simulink model "p560_jacobiano_ciclico_sp"  (R2020b)
settings: Solver=VariableStepAuto  StartTime=0.0  StopTime=50  RelTol=1e-3
values from neighbouring files (symbols this model uses):
  fr = 1    [init.m]
undefined symbols (not defined in the file or in its folder): DiscIntNeverNeededParam, qn
libraries: roblocks x6
settings Model: Creator=Valentina  LastModifiedBy=Valentina

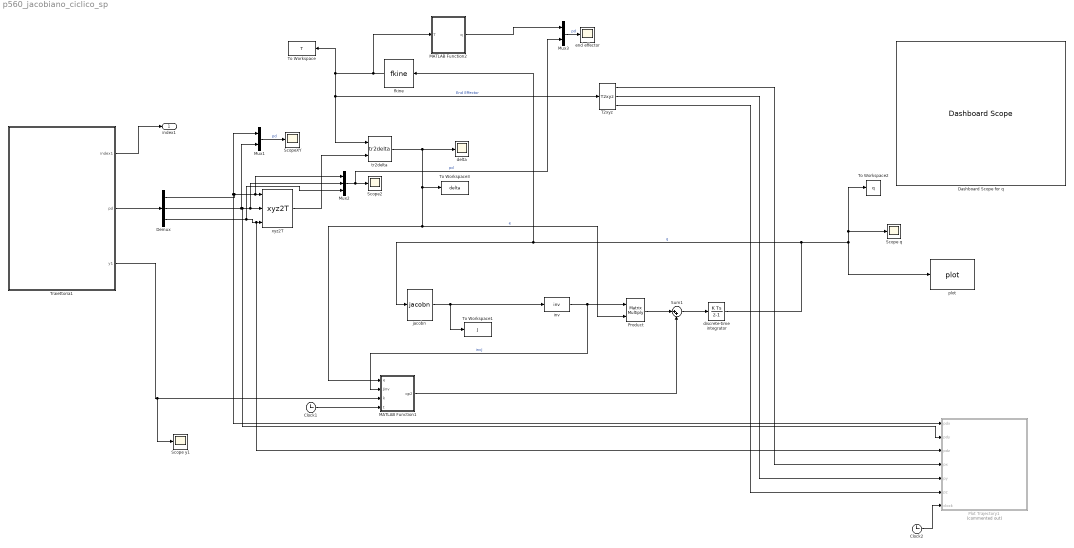
== system p560_jacobiano_ciclico_sp ==
  Clock1 : Clock
  Clock2 : Clock
  Dashboard Scope for q : DashboardScope
  Demux : Demux  Outputs=3
  MATLAB Function1 : MATLAB Function  Priority=6  TreatAsAtomicUnit=on  SystemSampleTime=2*pi/100
  MATLAB Function2 : MATLAB Function  Priority=6  TreatAsAtomicUnit=on
  Mux1 : Mux  Inputs=2
  Mux2 : Mux  Inputs=3
  Mux3 : Mux  Inputs=2
  Plot Trajectory1 : MATLAB Function  Commented=on  TreatAsAtomicUnit=on  SystemSampleTime=0.1
  Product : Product  Multiplication=Matrix(*)  InputSameDT=on  RndMeth=Zero  SaturateOnIntegerOverflow=on  OutDataTypeStr=Inherit: Same as first input
  Scope q : Scope
  Scope y1 : Scope
  Scope2 : Scope
  ScopeXY : Scope
  Sum1 : Sum  Inputs=|++
  T2xyz : roblocks/Toolbox/T2xyz
  To Workspace : ToWorkspace  VariableName=T  SampleTime=-1
  To Workspace1 : ToWorkspace  VariableName=J  SampleTime=-1
  To Workspace2 : ToWorkspace  VariableName=q  SampleTime=-1
  To Workspace3 : ToWorkspace  VariableName=delta  SampleTime=-1
  Traiettoria1 : Subsystem
  delta : Scope
  discrete-time integrator : DiscreteIntegrator  gainval=5  InitialCondition=qn  SampleTime=0.1  ICPrevOutput=DiscIntNeverNeededParam  ICPrevScaledInput=DiscIntNeverNeededParam
  end effector : Scope
  fkine : roblocks/Arm/fkine  robot=p560
  inv : MATLABFcn  MATLABFcn=inv  Output1D=off
  jacobn : roblocks/Arm/jacobn  robot=p560
  plot : roblocks/Arm/plot  robot=p560  fps=5  holdplot=on
  tr2delta : roblocks/Toolbox/tr2delta
  xyz2T : roblocks/Toolbox/xyz2T
  index1 : Outport
  wires:
  T2xyz/3 -> Plot Trajectory1/6(pz)
  Demux/1 -> Mux1/1, Plot Trajectory1/1(pdx), Mux2/1, xyz2T/1
  T2xyz/1 -> Plot Trajectory1/4(px)
  Clock2/1 -> Plot Trajectory1/7(clock)
  fkine/1 -> MATLAB Function2/1(T), To Workspace/1, tr2delta/1, T2xyz/1  "End Effector"
  T2xyz/2 -> Plot Trajectory1/5(py)
  tr2delta/1 -> delta/1, To Workspace3/1, Product/2, MATLAB Function1/1(e)  "e"
  Mux1/1 -> ScopeXY/1  "pd"
  MATLAB Function1/1(qp2) -> Sum1/2
  Demux/2 -> Mux1/2, Plot Trajectory1/2(pdy), Mux2/2, xyz2T/2
  jacobn/1 -> To Workspace1/1, inv/1
  xyz2T/1 -> tr2delta/2
  Sum1/1 -> discrete-time integrator/1
  discrete-time integrator/1 -> fkine/1, jacobn/1, plot/1, Scope q/1, To Workspace2/1  "q"
  Clock1/1 -> MATLAB Function1/4(t)
  inv/1 -> MATLAB Function1/2(Jinv), Product/1  "invJ"
  Product/1 -> Sum1/1
  Demux/3 -> Mux2/3, Plot Trajectory1/3(pdz), xyz2T/3
  Traiettoria1/2(pd) -> Demux/1
  Traiettoria1/1(index1) -> index1/1
  Traiettoria1/3(y1) -> Scope y1/1, MATLAB Function1/3(k)
  Mux2/1 -> Mux3/2, Scope2/1  "pd"
  Mux3/1 -> end effector/1  "pd"
  MATLAB Function2/1(q) -> Mux3/1

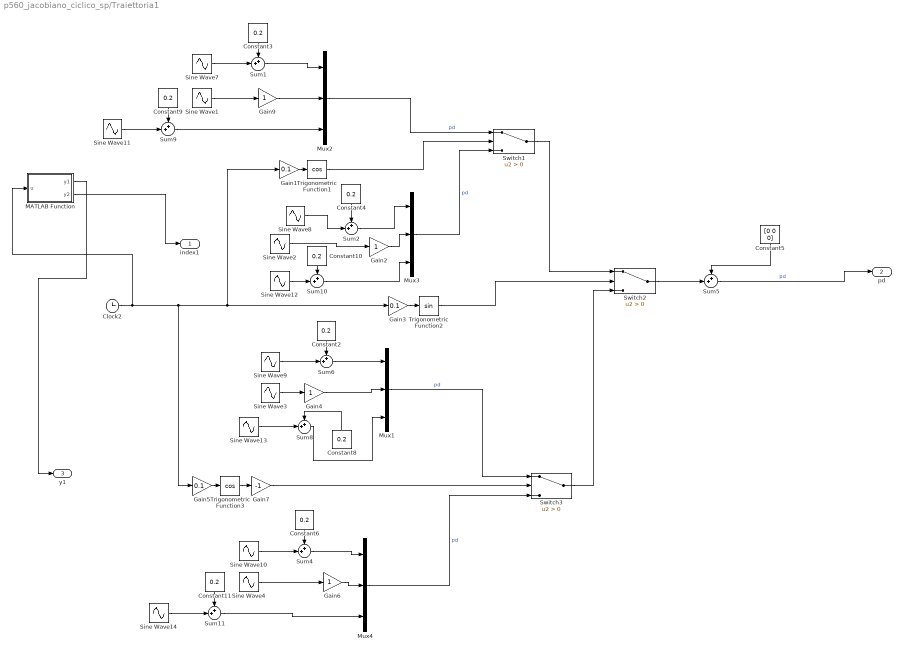
== system p560_jacobiano_ciclico_sp/Traiettoria1 ==
  Clock2 : Clock
  Constant{2..4,6,8..11} (8 alike) : Constant  Value=0.2
  Constant5 : Constant  Value=[0 0 0]
  Gain1 : Gain  Gain=0.1
  Gain{2,4,6,9} (4 alike) : Gain
  Gain3 : Gain  Gain=0.1
  Gain5 : Gain  Gain=0.1
  Gain7 : Gain  Gain=-1
  MATLAB Function : MATLAB Function  TreatAsAtomicUnit=on  SystemSampleTime=2*pi/100
  Mux{1..4} (4 alike) : Mux  Inputs=3
  Sine Wave{1..4} (4 alike) : Sin  Amplitude=0.5  Frequency=fr  Phase=pi/2  SampleTime=0
  Sine Wave{7..10} (4 alike) : Sin  Amplitude=0.5  Frequency=fr  SampleTime=0
  Sine Wave{11..14} (4 alike) : Sin  Amplitude=0.2  Frequency=fr  SampleTime=0
  Sum{1..2,4..6,8..11} (9 alike) : Sum  Inputs=++|
  Switch1 : Switch  Criteria=u2 > Threshold
  Switch2 : Switch  Criteria=u2 > Threshold
  Switch3 : Switch  Criteria=u2 > Threshold
  Trigonometric Function1 : Trigonometry  Operator=cos
  Trigonometric Function2 : Trigonometry
  Trigonometric Function3 : Trigonometry  Operator=cos
  index1 : Outport
  pd : Outport  Port=2
  y1 : Outport  Port=3
  wires:
  Gain3/1 -> Trigonometric Function2/1
  Gain5/1 -> Trigonometric Function3/1
  Switch1/1 -> Switch2/1
  Gain1/1 -> Trigonometric Function1/1
  Switch3/1 -> Switch2/3
  Mux4/1 -> Switch3/3  "pd"
  Mux1/1 -> Switch3/1  "pd"
  Gain7/1 -> Switch3/2
  ? -> ?
  Mux2/1 -> Switch1/1  "pd"
  Trigonometric Function1/1 -> Switch1/2
  Clock2/1 -> MATLAB Function/1(u), Gain1/1, Gain3/1, Gain5/1
  Sum5/1 -> pd/1  "pd"
  MATLAB Function/2(y2) -> index1/1
  MATLAB Function/1(y1) -> y1/1
  Trigonometric Function3/1 -> Gain7/1
  Trigonometric Function2/1 -> Switch2/2
  Mux3/1 -> Switch1/3  "pd"
  Constant5/1 -> Sum5/1
  ? -> ?
  Sum1/1 -> Mux2/1
  Constant3/1 -> Sum1/1
  Sine Wave1/1 -> Gain9/1
  Sine Wave7/1 -> Sum1/2
  Sum2/1 -> Mux3/1
  Constant4/1 -> Sum2/1
  Sine Wave2/1 -> Gain2/1
  Sine Wave8/1 -> Sum2/2
  Gain2/1 -> Mux3/2
  Sum6/1 -> Mux1/1
  Constant2/1 -> Sum6/1
  Sine Wave9/1 -> Sum6/2
  Sum4/1 -> Mux4/1
  Constant6/1 -> Sum4/1
  Sine Wave4/1 -> Gain6/1
  Sine Wave10/1 -> Sum4/2
  Gain6/1 -> Mux4/2
  Sine Wave3/1 -> Gain4/1
  Gain4/1 -> Mux1/2
  Gain9/1 -> Mux2/2
  Constant9/1 -> Sum9/1
  Sum9/1 -> Mux2/3
  Sine Wave11/1 -> Sum9/2
  Constant10/1 -> Sum10/1
  Sum10/1 -> Mux3/3
  Sine Wave12/1 -> Sum10/2
  Constant8/1 -> Sum8/1
  Sum8/1 -> Mux1/3
  Sine Wave13/1 -> Sum8/2
  Constant11/1 -> Sum11/1
  Sum11/1 -> Mux4/3
  Sine Wave14/1 -> Sum11/2
  Switch2/1 -> Sum5/2

== matlab function p560_jacobiano_ciclico_sp/Plot Trajectory1 ==
  settings: updateMethod=DISCRETE
  data: pdx input; pdy input; pdz input; px input; py input; pz input; clock input
function PlotTraiettoria(pdx,pdy,pdz,px,py,pz, clock)

eml.extrinsic('findobj','get','set','figure','clf',...
              'hold','delete','plot','axis','grid',...
              'hggroup','quiver','drawnow');
          
persistent target;
% persistent chain;
% persistent velocity;
% persistent chain2;
persistent i;
persistent k;

persistent obiettivo;


n=1;


if isempty(target)
    target=zeros(n,1);
    i=0;
    
end

if isempty(obiettivo)
    obiettivo=zeros(n,1);
    k=0;
end


i=i+1;
if i>n
    i=1;
end

k=k+1;
if k>n
    k=1;
end

%           
% pex=[0;...
%     cos(theta1);...
%     cos(theta1)+cos(theta1+theta2);...
%     cos(theta1)+cos(theta1+theta2)+cos(theta1+theta2+theta3)];
% 
% pey=[0;...
%     sin(theta1);...
%     sin(theta1)+sin(theta1+theta2);...
%     sin(theta1)+sin(theta1+theta2)+sin(theta1+theta2+theta3)];
% 
% 
% pex2=[0;...
%     cos(th1);...
%     cos(th1)+cos(th1+th2);...
%     cos(th1)+cos(th1+th2)+cos(th1+th2+th3)];
% 
% pey2=[0;...
%     sin(th1);...
%     sin(th1)+sin(th1+th2);...
%     sin(th1)+sin(th1+th2)+sin(th1+th2+th3)];
% 
% 
%           
foundFig=findobj('Tag','trajScope');
    
%if ~isempty(foundFig) & (clock==1)
%    delete(foundFig)
%    foundFig=findobj('Tag','trajScope');  
%end


 if isempty(foundFig)
    fig=figure('Color','white');
%    clf(fig);
    set(fig,'Name','Trajectory');
    set(fig,'DoubleBuffer','on','Tag','trajScope');
    set(fig,'Renderer','painters');
    hold('on');
    hax=get(fig,'CurrentAxes');
    set(hax,'DrawMode','fast','Box','off');    
    
    target(i)=plot3(hax,pdx,pdy,pdz,'bo','MarkerFaceColor','#4DBEEE');
  
 else
    hax=get(foundFig,'CurrentAxes');

end
% 
j=i-(n-1);
if j<=0
    j=j+n;
end

if target(j)~=0
    delete(target(j));
end

% draw the desired point
target(i)=plot3(pdx,pdy,pdz,'bo','MarkerFaceColor','#4DBEEE');
target(k)=plot3(px,py,pz,'rh','MarkerFaceColor','r');


grid('on');
axis([-1 1 -1 1 -1 1])
drawnow;

== matlab function p560_jacobiano_ciclico_sp/Traiettoria1/MATLAB Function ==
  data: u input; y1 output; y2 output
function [y1,y2] = fcn(u)

fr=1;
y1 = floor(100.*mod(fr.*u,(2*pi)) /(2*pi))+1;
y2 = floor(0.3*u/(2*pi));

== matlab function p560_jacobiano_ciclico_sp/MATLAB Function2 ==
  settings: updateMethod=DISCRETE
  data: T input; q output
function q = fcn(T)

q=zeros(3,1);
q(1)=T(1,4);
q(2)=T(2,4);
q(3)=T(3,4);

== matlab function p560_jacobiano_ciclico_sp/MATLAB Function1 ==
  settings: updateMethod=DISCRETE
  data: e input; Jinv input; qp2 output size=6; k input; t input
function qp2 = fcn(e,Jinv,k, t)

persistent f_v
persistent e_v
persistent last_k

n=100;

if isempty(last_k)
    last_k=-1;
end


if isempty(f_v)
    f_v=zeros(n,6);
end
   
if isempty(e_v)
    e_v=zeros(n,6);
end


if k~=last_k
%   
     %disp(k)
     last_k=k;
     
     if t<8*pi
        f_v(k,:)=0.6.*f_v(k,:); %+(Jinv*e_v(k,:)')';
     else
        f_v(k,:)=0.99.*f_v(k,:)+0.5*(Jinv*e_v(k,:)')';
     end
     
     
     e_v(k,:)=e';
%     
%  
end


qp2=f_v(k,:)';
